simulink model "tarea_ejercicio2_02_02_17"  (R2013a)
settings: Solver=ode45  StartTime=0.0  StopTime=20  RelTol=1e-3
libraries: dspsrcs4 x1, simulink x1
settings Model: Creator=Miguel  LastModifiedBy=Miguel

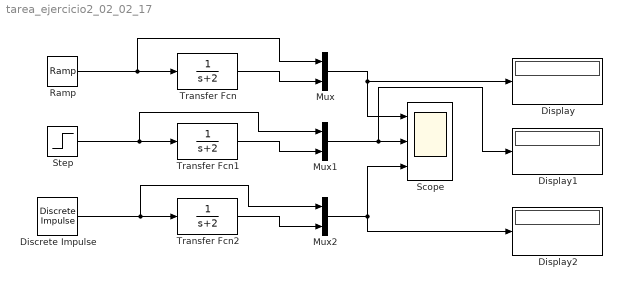
== system tarea_ejercicio2_02_02_17 ==
  Discrete Impulse : dspsrcs4/Discrete  Impulse  Delay=0  SampleTime=1  FrameSample=1  dataType=double  isSigned=on  wordLen=16  udDataType=sfix(16)  fracBitsMode=Best precision  numFracBits=15  OutDataTypeStr=double  LastOutDataTypeStr=double
  Display : Display
  Display1 : Display
  Display2 : Display
  Mux : Mux  Inputs=2
  Mux1 : Mux  Inputs=2
  Mux2 : Mux  Inputs=2
  Ramp : simulink/Sources/Ramp  slope=1  start=0  X0=0
  Scope : Scope  NumInputPorts=3
      settings: TickLabels=on  ShowLegends=on  YMin=-5~-5~-5  YMax=5~5~5
  Step : Step  SampleTime=0
  Transfer Fcn : TransferFcn  Denominator=[1 2]
  Transfer Fcn1 : TransferFcn  Denominator=[1 2]
  Transfer Fcn2 : TransferFcn  Denominator=[1 2]
  wires:
  Ramp/1 -> Mux/1, Transfer Fcn/1
  Step/1 -> Mux1/1, Transfer Fcn1/1
  Discrete Impulse/1 -> Mux2/1, Transfer Fcn2/1
  Transfer Fcn2/1 -> Mux2/2
  Transfer Fcn1/1 -> Mux1/2
  Transfer Fcn/1 -> Mux/2
  Mux1/1 -> Display1/1, Scope/2
  Mux/1 -> Display/1, Scope/1
  Mux2/1 -> Display2/1, Scope/3
